simulink model "EKMSL"  (R2020b)
settings: Solver=VariableStepAuto  StartTime=0.0  StopTime=10.0  MaxStep=EKM.T_ABS/25  RelTol=1e-4
undefined symbols (not defined in the file or in its folder): EKM
libraries: simulink x1
settings Model: Creator=Szalay  LastModifiedBy=Szalay

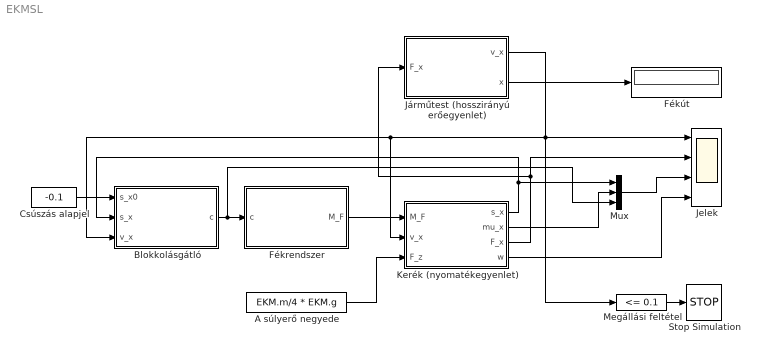
== system EKMSL ==
  A súlyerő negyede : Constant  Value=EKM.m/4 * EKM.g
  Blokkolásgátló : Subsystem
  Csúszás alapjel : Constant  Value=-0.1
  Fékrendszer : Subsystem
  Fékút : Display
  Jelek : Scope  NumInputPorts=4
  Járműtest (hosszirányú erőegyenlet) : Subsystem
  Kerék (nyomatékegyenlet) : Subsystem
  Megállási feltétel : simulink/Logic and Bit Operations/Compare To Constant  relop=<=  const=0.1  OutDataTypeStr=boolean
  Mux : Mux  Inputs=3
  Stop Simulation : Stop
  wires:
  Kerék (nyomatékegyenlet)/3(F_x) -> Jelek/2, Járműtest (hosszirányú erőegyenlet)/1(F_x)
  Járműtest (hosszirányú erőegyenlet)/1(v_x) -> Megállási feltétel/1, Blokkolásgátló/3(v_x), Kerék (nyomatékegyenlet)/2(v_x), Jelek/1
  A súlyerő negyede/1 -> Kerék (nyomatékegyenlet)/3(F_z)
  Kerék (nyomatékegyenlet)/1(s_x) -> Blokkolásgátló/2(s_x), Mux/1
  Mux/1 -> Jelek/3
  Kerék (nyomatékegyenlet)/2(mu_x) -> Mux/2
  Kerék (nyomatékegyenlet)/4(w) -> Jelek/4
  Megállási feltétel/1 -> Stop Simulation/1
  Járműtest (hosszirányú erőegyenlet)/2(x) -> Fékút/1
  Fékrendszer/1(M_F) -> Kerék (nyomatékegyenlet)/1(M_F)
  Blokkolásgátló/1(c) -> Mux/3, Fékrendszer/1(c)
  Csúszás alapjel/1 -> Blokkolásgátló/1(s_x0)

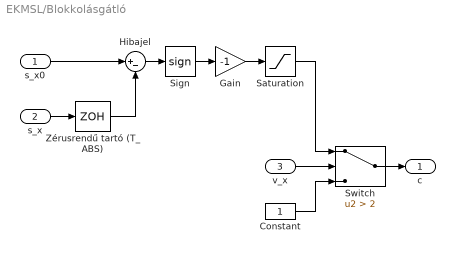
== system EKMSL/Blokkolásgátló ==
  s_x0 : Inport
  s_x : Inport  Port=2
  v_x : Inport  Port=3
  Constant : Constant
  Gain : Gain  Gain=-1
  Hibajel : Sum  Inputs=|+-
  Saturation : Saturate  UpperLimit=1  LowerLimit=0
  Sign : Signum
  Switch : Switch  Criteria=u2 > Threshold  Threshold=2
  Zérusrendű tartó (T_ABS) : ZeroOrderHold  SampleTime=EKM.T_ABS
  c : Outport
  wires:
  s_x/1 -> Zérusrendű tartó (T_ABS)/1
  s_x0/1 -> Hibajel/1
  Zérusrendű tartó (T_ABS)/1 -> Hibajel/2
  Hibajel/1 -> Sign/1
  Sign/1 -> Gain/1
  Gain/1 -> Saturation/1
  Switch/1 -> c/1
  Saturation/1 -> Switch/1
  v_x/1 -> Switch/2
  Constant/1 -> Switch/3

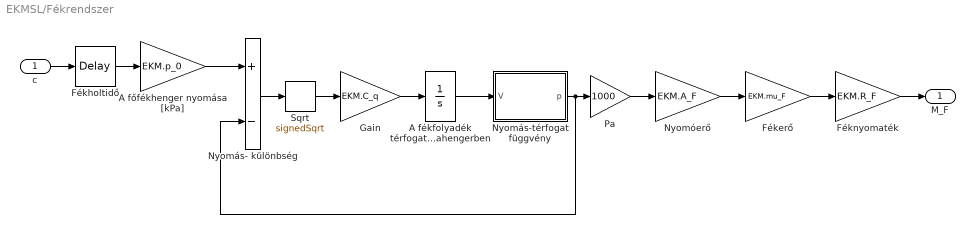
== system EKMSL/Fékrendszer ==
  c : Inport
  A fékfolyadék térfogata a fékmunkahengerben : Integrator  LimitOutput=on  LowerSaturationLimit=0
  A főfékhenger nyomása [kPa] : Gain  Gain=EKM.p_0
  Fékerő : Gain  Gain=EKM.mu_F
  Fékholtidő : TransportDelay  DelayTime=EKM.T_D
  Féknyomaték : Gain  Gain=EKM.R_F
  Gain : Gain  Gain=EKM.C_q
  Nyomás- különbség : Sum  Inputs=+-
  Nyomás-térfogat függvény : MATLAB Function  TreatAsAtomicUnit=on
  Nyomóerő : Gain  Gain=EKM.A_F
  Pa : Gain  Gain=1000
  Sqrt : Sqrt  Operator=signedSqrt  SaturateOnIntegerOverflow=on
  M_F : Outport
  wires:
  c/1 -> Fékholtidő/1
  Fékholtidő/1 -> A főfékhenger nyomása [kPa]/1
  A főfékhenger nyomása [kPa]/1 -> Nyomás- különbség/1
  Nyomás- különbség/1 -> Sqrt/1
  Sqrt/1 -> Gain/1
  Gain/1 -> A fékfolyadék térfogata a fékmunkahengerben/1
  A fékfolyadék térfogata a fékmunkahengerben/1 -> Nyomás-térfogat függvény/1(V)
  Nyomás-térfogat függvény/1(p) -> Nyomás- különbség/2, Pa/1
  Pa/1 -> Nyomóerő/1
  Nyomóerő/1 -> Fékerő/1
  Fékerő/1 -> Féknyomaték/1
  Féknyomaték/1 -> M_F/1

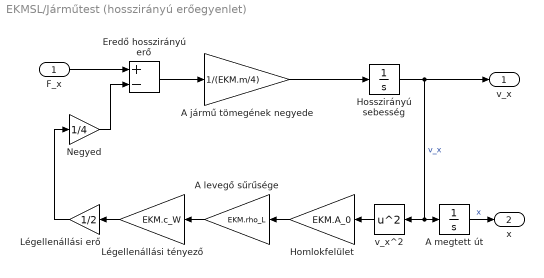
== system EKMSL/Járműtest (hosszirányú erőegyenlet) ==
  F_x : Inport
  A jármű tömegének negyede : Gain  Gain=1/(EKM.m/4)
  A levegő sűrűsége : Gain  Gain=EKM.rho_L
  A megtett út : Integrator
  Eredő hosszirányú erő : Sum  Inputs=+-
  Homlokfelület : Gain  Gain=EKM.A_0
  Hosszirányú sebesség : Integrator  InitialCondition=20
  Légellenállási erő : Gain  Gain=1/2
  Légellenállási tényező : Gain  Gain=EKM.c_W
  Negyed : Gain  Gain=1/4
  v_x^2 : Math  Operator=square  SaturateOnIntegerOverflow=on
  v_x : Outport
  x : Outport  Port=2
  wires:
  Hosszirányú sebesség/1 -> v_x/1, v_x^2/1, A megtett út/1  "v_x"
  A megtett út/1 -> x/1  "x"
  v_x^2/1 -> Homlokfelület/1
  Homlokfelület/1 -> A levegő sűrűsége/1
  A levegő sűrűsége/1 -> Légellenállási tényező/1
  Légellenállási tényező/1 -> Légellenállási erő/1
  Légellenállási erő/1 -> Negyed/1
  F_x/1 -> Eredő hosszirányú erő/1
  Negyed/1 -> Eredő hosszirányú erő/2
  Eredő hosszirányú erő/1 -> A jármű tömegének negyede/1
  A jármű tömegének negyede/1 -> Hosszirányú sebesség/1

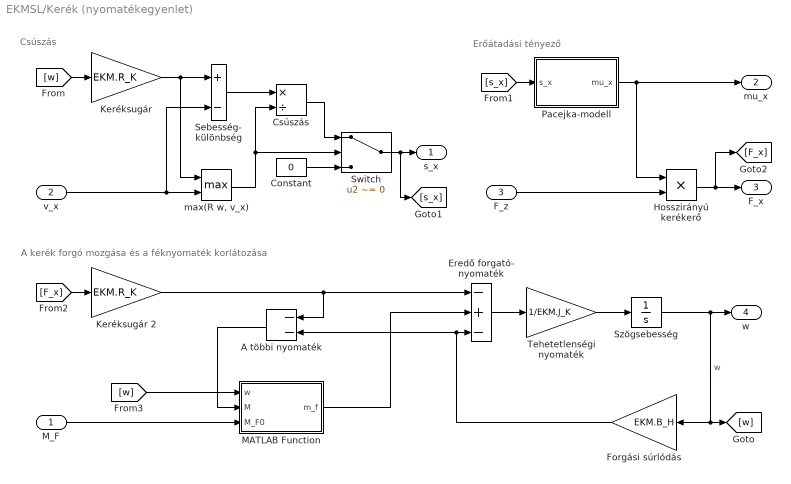
== system EKMSL/Kerék (nyomatékegyenlet) ==
  note: A kerék forgó mozgása és a féknyomaték korlátozása
  note: Erőátadási tényező
  note: Csúszás
  M_F : Inport
  v_x : Inport  Port=2
  F_z : Inport  Port=3
  A többi nyomaték : Sum  Inputs=--
  Constant : Constant  Value=0
  Csúszás : Product  Inputs=*/
  Eredő forgató- nyomaték : Sum  Inputs=-+-
  Forgási súrlódás : Gain  Gain=EKM.B_H
  Hosszirányú kerékerő : Product
  Keréksugár : Gain  Gain=EKM.R_K
  Keréksugár 2 : Gain  Gain=EKM.R_K
  MATLAB Function : MATLAB Function  TreatAsAtomicUnit=on
  Pacejka-modell : MATLAB Function  TreatAsAtomicUnit=on
  Sebesség- különbség : Sum  Inputs=+-
  Switch : Switch  Criteria=u2 ~= 0
  Szögsebesség : Integrator  InitialCondition=20/EKM.R_K  LimitOutput=on  LowerSaturationLimit=0
  Tehetetlenségi nyomaték : Gain  Gain=1/EKM.J_K
  "max(R w, v_x)" : MinMax  Function=max  Inputs=2
  s_x : Outport
  mu_x : Outport  Port=2
  F_x : Outport  Port=3
  w : Outport  Port=4
  wires:
  Szögsebesség/1 -> [w], Forgási súrlódás/1, w/1  "w"
  [w] -> Keréksugár/1
  Keréksugár/1 -> "max(R w, v_x)"/1, Sebesség- különbség/1
  v_x/1 -> "max(R w, v_x)"/2, Sebesség- különbség/2
  Sebesség- különbség/1 -> Csúszás/1
  "max(R w, v_x)"/1 -> Switch/2, Csúszás/2
  Csúszás/1 -> Switch/1
  Constant/1 -> Switch/3
  Switch/1 -> [s_x], s_x/1
  F_z/1 -> Hosszirányú kerékerő/2
  Hosszirányú kerékerő/1 -> [F_x], F_x/1
  [s_x] -> Pacejka-modell/1(s_x)
  Pacejka-modell/1(mu_x) -> Hosszirányú kerékerő/1, mu_x/1
  Tehetetlenségi nyomaték/1 -> Szögsebesség/1
  Eredő forgató- nyomaték/1 -> Tehetetlenségi nyomaték/1
  Forgási súrlódás/1 -> A többi nyomaték/2, Eredő forgató- nyomaték/3
  [F_x] -> Keréksugár 2/1
  Keréksugár 2/1 -> A többi nyomaték/1, Eredő forgató- nyomaték/1
  M_F/1 -> MATLAB Function/3(M_F0)
  [w] -> MATLAB Function/1(w)
  A többi nyomaték/1 -> MATLAB Function/2(M)
  MATLAB Function/1(m_f) -> Eredő forgató- nyomaték/2

== matlab function EKMSL/Kerék (nyomatékegyenlet)/Pacejka-modell ==
  data: s_x input; mu_x output
function mu_x = Pacejka(s_x)

mu_x = EKM.Pacejka(s_x);

== matlab function EKMSL/Fékrendszer/Nyomás-térfogat függvény ==
  data: V input; p output
function p = Brake(V)

p = EKM.BrakePressureModel(V);

== matlab function EKMSL/Kerék (nyomatékegyenlet)/MATLAB Function ==
  data: w input; m_f output; M input; M_F0 input
function m_f = M_F(w, M, M_F0)

m_f = EKM.M_F(w, M, M_F0);
